simulink model "tong_hop_truc_tiep_2022"  (R2022a)
settings: Solver=ode15s  StartTime=0.0  StopTime=20000  MaxStep=20000.0  RelTol=1e-3
values from neighbouring files (symbols this model uses):
  Kc = Tp_obj / (Kp_obj * Tc)    [tong_hop_truc_tiep.m]
  Kff = 1/KL    [tong_hop_truc_tiep.m]
  Ki_sim = Kc / Ti    [tong_hop_truc_tiep.m]
undefined symbols (not defined in the file or in its folder): den_D12, den_D21, num_D12, num_D21
libraries: simulink x2, slpidlib x2
settings Model: Creator=PC  LastModifiedBy=Moderator
settings SolverCC: ZeroCrossAlgorithm=Adaptive
settings DebuggingCC: IgnoredZcDiagnostic=none
settings ModelReferenceCC: EnableRefExpFcnMdlSchedulingChecks=off
settings RTWCC: Description=Generic Real-Time Target  GPUComputeCapability=5.0

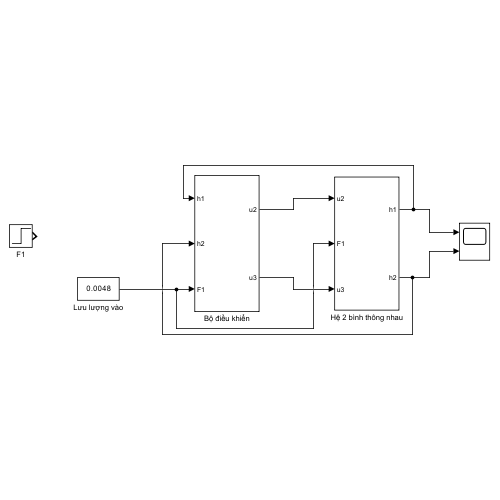
[thumbnail: Simulink's stored preview of the top-level diagram]
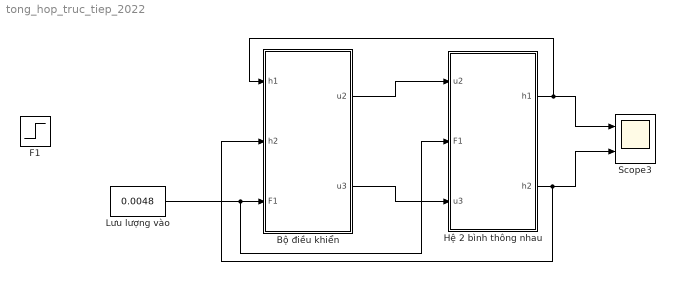
== system tong_hop_truc_tiep_2022 ==
  Bộ điều khiển : Subsystem
  F1 : Step  Time=10000  Before=0.0048  After=0.007  SampleTime=0
  Hệ 2 bình thông nhau : Subsystem
  Lưu lượng vào : Constant  Value=0.0048
  Scope3 : Scope  NumInputPorts=2
  wires:
  Bộ điều khiển/2(u3) -> Hệ 2 bình thông nhau/3(u3)
  Bộ điều khiển/1(u2) -> Hệ 2 bình thông nhau/1(u2)
  Hệ 2 bình thông nhau/1(h1) -> Bộ điều khiển/1(h1), Scope3/1
  Hệ 2 bình thông nhau/2(h2) -> Scope3/2, Bộ điều khiển/2(h2)
  Lưu lượng vào/1 -> Hệ 2 bình thông nhau/2(F1), Bộ điều khiển/3(F1)

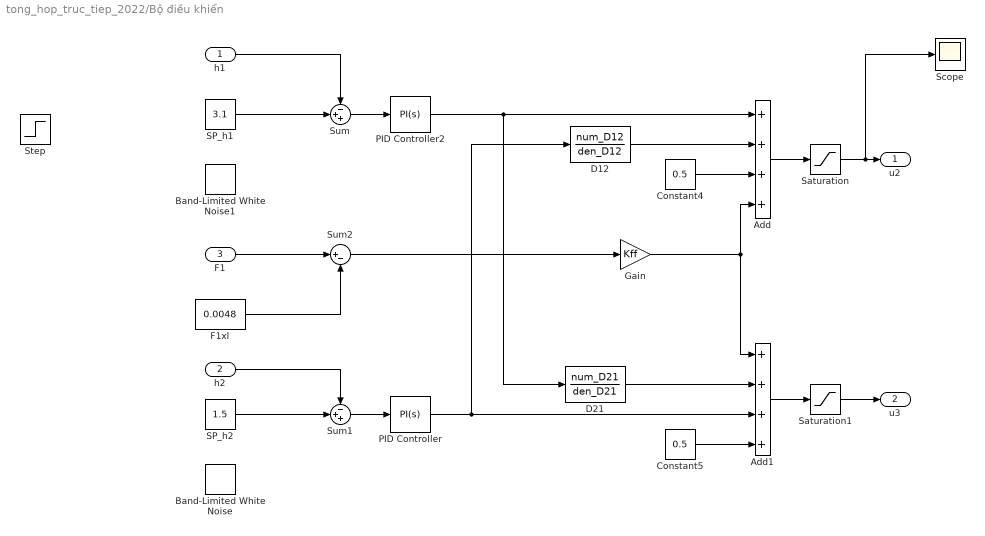
== system tong_hop_truc_tiep_2022/Bộ điều khiển ==
  h1 : Inport
  h2 : Inport  Port=2
  F1 : Inport  Port=3
  Add : Sum  Inputs=++++
  Add1 : Sum  Inputs=++++
  Band-Limited White Noise : simulink/Sources/Band-Limited White Noise  Cov=[0.0001]  Ts=0.1  seed=[23341]
  Band-Limited White Noise1 : simulink/Sources/Band-Limited White Noise  Cov=[0.0001]  Ts=0.1  seed=[23341]
  Constant4 : Constant  Value=0.5
  Constant5 : Constant  Value=0.5
  D12 : TransferFcn  Numerator=num_D12  Denominator=den_D12
  D21 : TransferFcn  Numerator=num_D21  Denominator=den_D21
  F1xl : Constant  Value=0.0048
  Gain : Gain  Gain=Kff
  PID Controller : slpidlib/PID Controller  Controller=PI  Form=Parallel  TimeDomain=Continuous-time  UseExternalTs=off  SampleTime=-1  IntegratorMethod=Forward Euler  FilterMethod=Forward Euler  ControllerParametersSource=internal  P=Kc  I=Ki_sim  UseKiTs=off  D=0  N=100  UseFilter=on  TunerSelectOption=Transfer Function Based (PID Tuner App)  InitialConditionSource=internal  InitialConditionForIntegrator=0  InitialConditionForFilter=0  DifferentiatorICPrevScaledInput=0  ExternalReset=none  TrackingMode=off  Kt=1  LimitOutput=on  SatLimitsSource=internal  UpperSaturationLimit=0.5  LowerSaturationLimit=-0.5  LinearizeAsGain=on  AntiWindupMode=clamping  Kb=1  POutMin=[]  POutMax=[]  IOutMin=[]  IOutMax=[]  DOutMin=[]  DOutMax=[]  NOutMin=[]  NOutMax=[]  SumOutMin=[]  SumOutMax=[]  SaturationOutMin=[]  SaturationOutMax=[]  PParamMin=[]  PParamMax=[]  IParamMin=[]  IParamMax=[]  DParamMin=[]  DParamMax=[]  NParamMin=[]  NParamMax=[]  KbParamMin=[]  KbParamMax=[]  KtParamMin=[]  KtParamMax=[]  KbOutMin=[]  KbOutMax=[]  KtOutMin=[]  KtOutMax=[]  IntegratorOutMin=[]  IntegratorOutMax=[]  FilterOutMin=[]  FilterOutMax=[]  SumI1OutMin=[]  SumI1OutMax=[]  SumI2OutMin=[]  SumI2OutMax=[]  SumI3OutMin=[]  SumI3OutMax=[]  SumI4OutMin=[]  SumI4OutMax=[]  SumDOutMin=[]  SumDOutMax=[]  DifferentiatorOutMin=[]  DifferentiatorOutMax=[]  FilterDiffOutCoefMin=[]  FilterDiffOutCoefMax=[]  ReciprocalOutMin=[]  ReciprocalOutMax=[]  SumDenOutMin=[]  SumDenOutMax=[]  SumNumOutMin=[]  SumNumOutMax=[]  DivideOutMin=[]  DivideOutMax=[]  UdiffTsProdOutMin=[]  UdiffTsProdOutMax=[]  NTsProdOutMin=[]  NTsProdOutMax=[]  UintegralTsProdOutMin=[]  UintegralTsProdOutMax=[]  UngainTsProdOutMin=[]  UngainTsProdOutMax=[]  IntegratorContinuousStateAttributes=''  IntegratorStateMustResolveToSignalObject=off  IntegratorRTWStateStorageClass=Auto  FilterContinuousStateAttributes=''  FilterStateMustResolveToSignalObject=off  FilterRTWStateStorageClass=Auto  ParallelPVariant=InternalParameters  IdealPVariant=Disabled  IVariant=InternalParameters  DVariant=Disabled  IntegratorVariant=Continuous  SatVariant=Enabled  AWVariant=ContClampingParallel  PCopyVariant=Disabled  TRVariant=Disabled  FdbkBlocksVariant=Forward  IdealPFdbkVariant=Disabled  SatFdbkVariant=Disabled  DerivativeFilterVariant=Disabled  NVariant=Disabled  NCopyVariant=Disabled_SignalSpec  FilterICVariant=Disabled  IntegratorICVariant=InternalICs  ExternalResetVariant=Disabled  TRSumVariant=Passthrough  SumFdbkVariant=Disabled  SumVariant=Sum_PI  TsampFilterVariant=InternalTs  TsampNgainVariant=Passthrough  TsampIntegralVariant=Disabled_SignalSpec  ExternalSaturationOutDataTypeStr=Inherit: Same as second input
  PID Controller2 : slpidlib/PID Controller  Controller=PI  Form=Parallel  TimeDomain=Continuous-time  UseExternalTs=off  SampleTime=-1  IntegratorMethod=Forward Euler  FilterMethod=Forward Euler  ControllerParametersSource=internal  P=Kc  I=Ki_sim  UseKiTs=off  D=0  N=100  UseFilter=on  TunerSelectOption=Transfer Function Based (PID Tuner App)  InitialConditionSource=internal  InitialConditionForIntegrator=0  InitialConditionForFilter=0  DifferentiatorICPrevScaledInput=0  ExternalReset=none  TrackingMode=off  Kt=1  LimitOutput=on  SatLimitsSource=internal  UpperSaturationLimit=0.5  LowerSaturationLimit=-0.5  LinearizeAsGain=on  AntiWindupMode=clamping  Kb=1  POutMin=[]  POutMax=[]  IOutMin=[]  IOutMax=[]  DOutMin=[]  DOutMax=[]  NOutMin=[]  NOutMax=[]  SumOutMin=[]  SumOutMax=[]  SaturationOutMin=[]  SaturationOutMax=[]  PParamMin=[]  PParamMax=[]  IParamMin=[]  IParamMax=[]  DParamMin=[]  DParamMax=[]  NParamMin=[]  NParamMax=[]  KbParamMin=[]  KbParamMax=[]  KtParamMin=[]  KtParamMax=[]  KbOutMin=[]  KbOutMax=[]  KtOutMin=[]  KtOutMax=[]  IntegratorOutMin=[]  IntegratorOutMax=[]  FilterOutMin=[]  FilterOutMax=[]  SumI1OutMin=[]  SumI1OutMax=[]  SumI2OutMin=[]  SumI2OutMax=[]  SumI3OutMin=[]  SumI3OutMax=[]  SumI4OutMin=[]  SumI4OutMax=[]  SumDOutMin=[]  SumDOutMax=[]  DifferentiatorOutMin=[]  DifferentiatorOutMax=[]  FilterDiffOutCoefMin=[]  FilterDiffOutCoefMax=[]  ReciprocalOutMin=[]  ReciprocalOutMax=[]  SumDenOutMin=[]  SumDenOutMax=[]  SumNumOutMin=[]  SumNumOutMax=[]  DivideOutMin=[]  DivideOutMax=[]  UdiffTsProdOutMin=[]  UdiffTsProdOutMax=[]  NTsProdOutMin=[]  NTsProdOutMax=[]  UintegralTsProdOutMin=[]  UintegralTsProdOutMax=[]  UngainTsProdOutMin=[]  UngainTsProdOutMax=[]  IntegratorContinuousStateAttributes=''  IntegratorStateMustResolveToSignalObject=off  IntegratorRTWStateStorageClass=Auto  FilterContinuousStateAttributes=''  FilterStateMustResolveToSignalObject=off  FilterRTWStateStorageClass=Auto  ParallelPVariant=InternalParameters  IdealPVariant=Disabled  IVariant=InternalParameters  DVariant=Disabled  IntegratorVariant=Continuous  SatVariant=Enabled  AWVariant=ContClampingParallel  PCopyVariant=Disabled  TRVariant=Disabled  FdbkBlocksVariant=Forward  IdealPFdbkVariant=Disabled  SatFdbkVariant=Disabled  DerivativeFilterVariant=Disabled  NVariant=Disabled  NCopyVariant=Disabled_SignalSpec  FilterICVariant=Disabled  IntegratorICVariant=InternalICs  ExternalResetVariant=Disabled  TRSumVariant=Passthrough  SumFdbkVariant=Disabled  SumVariant=Sum_PI  TsampFilterVariant=InternalTs  TsampNgainVariant=Passthrough  TsampIntegralVariant=Disabled_SignalSpec  ExternalSaturationOutDataTypeStr=Inherit: Same as second input
  SP_h1 : Constant  Value=3.1
  SP_h2 : Constant  Value=1.5
  Saturation : Saturate  UpperLimit=1  LowerLimit=0
  Saturation1 : Saturate  UpperLimit=1  LowerLimit=0
  Scope : Scope
  Step : Step  Time=10000  Before=3  After=3.1  SampleTime=0
  Sum : Sum  Inputs=-++
  Sum1 : Sum  Inputs=-++
  Sum2 : Sum  Inputs=|+-
  u2 : Outport
  u3 : Outport  Port=2
  wires:
  PID Controller2/1 -> D21/1, Add/1
  Constant4/1 -> Add/3
  Saturation/1 -> Scope/1, u2/1
  Sum1/1 -> PID Controller/1
  Add/1 -> Saturation/1
  Add1/1 -> Saturation1/1
  Sum/1 -> PID Controller2/1
  Saturation1/1 -> u3/1
  PID Controller/1 -> D12/1, Add1/3
  h2/1 -> Sum1/1
  h1/1 -> Sum/1
  SP_h2/1 -> Sum1/2
  Gain/1 -> Add1/1, Add/4
  F1/1 -> Sum2/1
  F1xl/1 -> Sum2/2
  Sum2/1 -> Gain/1
  Constant5/1 -> Add1/4
  SP_h1/1 -> Sum/2
  D12/1 -> Add/2
  D21/1 -> Add1/2

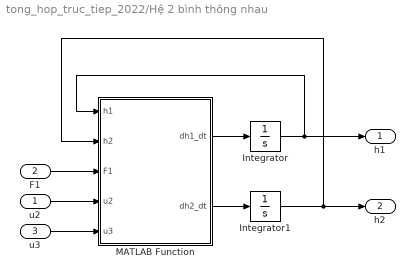
== system tong_hop_truc_tiep_2022/Hệ 2 bình thông nhau ==
  u2 : Inport
  F1 : Inport  Port=2
  u3 : Inport  Port=3
  Integrator : Integrator  InitialCondition=3
  Integrator1 : Integrator  InitialCondition=1.5
  MATLAB Function : MATLAB Function  TreatAsAtomicUnit=on
  h1 : Outport
  h2 : Outport  Port=2
  wires:
  MATLAB Function/2(dh2_dt) -> Integrator1/1
  Integrator1/1 -> MATLAB Function/2(h2), h2/1
  Integrator/1 -> h1/1, MATLAB Function/1(h1)
  MATLAB Function/1(dh1_dt) -> Integrator/1
  u2/1 -> MATLAB Function/4(u2)
  F1/1 -> MATLAB Function/3(F1)
  u3/1 -> MATLAB Function/5(u3)

== matlab function tong_hop_truc_tiep_2022/Hệ 2 bình thông nhau/MATLAB Function ==
  data: h1 input; dh1_dt output; h2 input; F1 input; u2 input; u3 input; dh2_dt output
function [dh1_dt, dh2_dt] = CoupledTanks(h1, h2, F1, u2, u3)
    % CÁC THÔNG SỐ VẬT LÝ CỦA HỆ THỐNG
    A1 = 1;       % Tiết diện bình 1 (m^2)
    A2 = 1;       % Tiết diện bình 2 (m^2)
    Cv = 0.0025;      % Hệ số lưu lượng của van
    g  = 9.81;      % Gia tốc trọng trường (m/s^2)
    gs = 1;         % Tỷ trọng của nước
    
    % RÀNG BUỘC VẬT LÝ (Chống lỗi toán học khi mô phỏng)
    % Không cho phép mức nước âm (nếu cạn thì = 0)
    if h1 < 0, h1 = 0; end
    if h2 < 0, h2 = 0; end
    
    % TÍNH TOÁN LƯU LƯỢNG QUA CÁC VAN (Theo phương trình vật lý)
    % Lưu lượng từ bình 1 sang bình 2 (F2)
    if h1 >= h2
        F2 = Cv * u2 * sqrt(abs((g * (h1 - h2)) / gs));
    else
        % Nếu h2 > h1, nước chảy ngược lại
        F2 = -Cv * u2 * sqrt(abs((g * (h2 - h1)) / gs)); 
    end
    
    % Lưu lượng xả từ bình 2 ra ngoài (F3)
    F3 = Cv * u3 * sqrt(abs((g * h2) / gs));
    
    % HỆ PHƯƠNG TRÌNH VI PHÂN (Tính đạo hàm của h1 và h2)
    dh1_dt = (F1 - F2) / A1;
    dh2_dt = (F2 - F3) / A2;
end
